simulink model "model_v1"  (R2019a)
settings: Solver=VariableStepAuto  StartTime=0.0  StopTime=10.0  RelTol=1e-3
values from neighbouring files (symbols this model uses):
  m = 200    [config_v1.m]
settings Model: Creator=jacoboffersen  LastModifiedBy=jacoboffersen

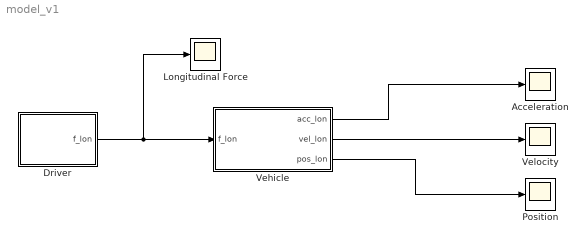
== system model_v1 ==
  Acceleration : Scope
  Driver : Subsystem
  Longitudinal Force : Scope
  Position : Scope
  Vehicle : Subsystem
  Velocity : Scope
  wires:
  Driver/1(f_lon) -> Longitudinal Force/1, Vehicle/1(f_lon)
  Vehicle/1(acc_lon) -> Acceleration/1
  Vehicle/2(vel_lon) -> Velocity/1
  Vehicle/3(pos_lon) -> Position/1

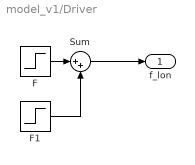
== system model_v1/Driver ==
  F : Step  Time=2  SampleTime=0
  F1 : Step  Time=4  After=-1  SampleTime=0
  Sum : Sum  Inputs=|++
  f_lon : Outport
  wires:
  F1/1 -> Sum/2
  F/1 -> Sum/1
  Sum/1 -> f_lon/1

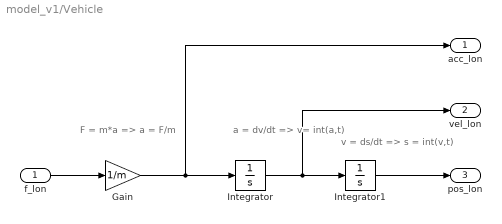
== system model_v1/Vehicle ==
  note: a = dv/dt =>
      | v= int(a,t)
  note: v = ds/dt =>
      | s = int(v,t)
  note: F = m*a =>
      | a = F/m
  f_lon : Inport
  Gain : Gain  Gain=1/m
  Integrator : Integrator
  Integrator1 : Integrator
  acc_lon : Outport
  vel_lon : Outport  Port=2
  pos_lon : Outport  Port=3
  wires:
  Integrator1/1 -> pos_lon/1
  Integrator/1 -> vel_lon/1, Integrator1/1
  Gain/1 -> acc_lon/1, Integrator/1
  f_lon/1 -> Gain/1
